simulink model "twoDOFmodel_side_wind_gust"  (R2020b)
settings: Solver=ode5  StartTime=0.0  StopTime=tf  FixedStep=dt  RelTol=1e-3
values from neighbouring files (symbols this model uses):
  I = 2500    [bicyclemodle_setp_disturbance_force_Param.m]    (also in bicyclemodle_stepParam.m; twoDOFmodel_side_wind_gust_Param.m)
  lw = -0.30    (= -0.3)    [twoDOFmodel_side_wind_gust_Param.m]
  m = 1500    [bicyclemodle_setp_disturbance_force_Param.m]    (also in bicyclemodle_stepParam.m; twoDOFmodel_side_wind_gust_Param.m)
  V = 80/3.6    (= 22.2222222222)    [bicyclemodle_setp_disturbance_force_Param.m]    (also in bicyclemodle_stepParam.m = 38.8888888889; twoDOFmodel_side_wind_gust_Param.m = 40)
  Yw = cy*0.5*p*s*(V*V+v*v)    (= 2066.58)    [twoDOFmodel_side_wind_gust_Param.m]
libraries: simulink x1
settings Model: Creator=Anson  LastModifiedBy=Anson

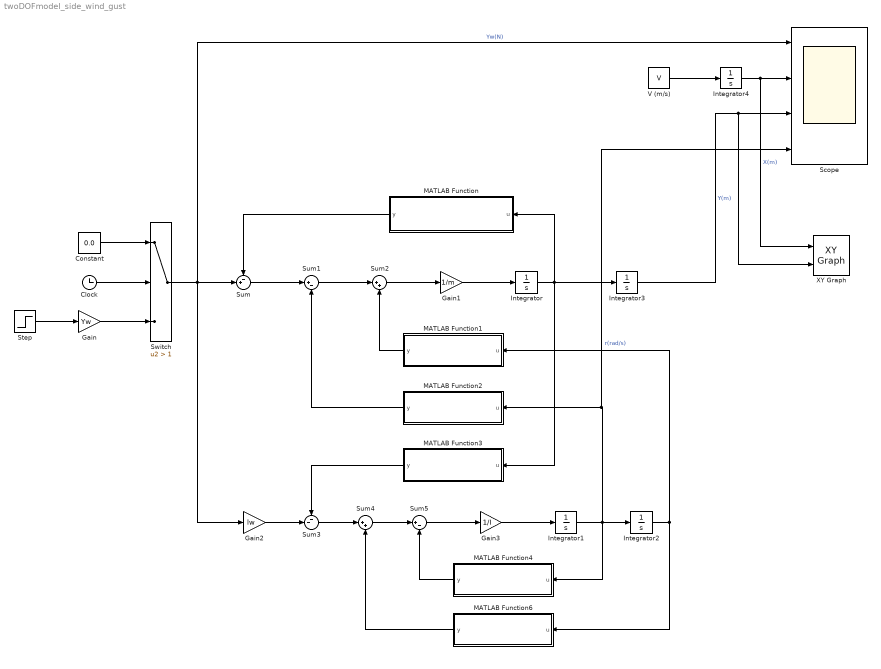
== system twoDOFmodel_side_wind_gust ==
  Clock : Clock
  Constant : Constant  Value=0.0
  Gain : Gain  Gain=Yw
  Gain1 : Gain  Gain=1/m
  Gain2 : Gain  Gain=lw
  Gain3 : Gain  Gain=1/I
  Integrator{,1..4} (5 alike) : Integrator
  MATLAB Function : MATLAB Function  TreatAsAtomicUnit=on
  MATLAB Function1 : MATLAB Function  TreatAsAtomicUnit=on
  MATLAB Function2 : MATLAB Function  TreatAsAtomicUnit=on
  MATLAB Function3 : MATLAB Function  TreatAsAtomicUnit=on
  MATLAB Function4 : MATLAB Function  TreatAsAtomicUnit=on
  MATLAB Function6 : MATLAB Function  TreatAsAtomicUnit=on
  Scope : Scope  NumInputPorts=4
  Step : Step  Time=0.5  SampleTime=0
  Sum : Sum  Inputs=-+|
  Sum1 : Sum  Inputs=|+-
  Sum2 : Sum  Inputs=|++
  Sum3 : Sum  Inputs=--|
  Sum4 : Sum  Inputs=|++
  Sum5 : Sum  Inputs=|+-
  Switch : Switch  Criteria=u2 > Threshold  Threshold=1
  V (m/s) : Constant  Value=V
  XY Graph : simulink/Sinks/XY Graph  xmin=-1  xmax=170  ymin=-1  ymax=3  st=-1
  wires:
  Step/1 -> Gain/1
  Clock/1 -> Switch/2
  Constant/1 -> Switch/1
  Gain/1 -> Switch/3
  Switch/1 -> Scope/1, Gain2/1, Sum/2  "Yw(N)"
  Sum1/1 -> Sum2/1
  Sum/1 -> Sum1/1
  Sum2/1 -> Gain1/1
  Gain1/1 -> Integrator/1
  Integrator/1 -> Integrator3/1, MATLAB Function3/1(u), MATLAB Function/1(u)
  MATLAB Function/1(y) -> Sum/1
  MATLAB Function1/1(y) -> Sum2/2
  MATLAB Function2/1(y) -> Sum1/2
  Gain2/1 -> Sum3/2
  MATLAB Function3/1(y) -> Sum3/1
  Sum3/1 -> Sum4/1
  MATLAB Function6/1(y) -> Sum4/2
  Sum4/1 -> Sum5/1
  MATLAB Function4/1(y) -> Sum5/2
  Sum5/1 -> Gain3/1
  Gain3/1 -> Integrator1/1
  Integrator1/1 -> Scope/4, MATLAB Function2/1(u), MATLAB Function4/1(u), Integrator2/1  "r(rad/s)"
  Integrator2/1 -> MATLAB Function6/1(u), MATLAB Function1/1(u)
  V (m/s)/1 -> Integrator4/1
  Integrator4/1 -> XY Graph/1, Scope/2  "X(m)"
  Integrator3/1 -> XY Graph/2, Scope/3  "Y(m)"

== matlab function twoDOFmodel_side_wind_gust/MATLAB Function ==
  data: u input; y output
function y = fcn(u)
Kf = 55000; % front cornering stiffness (N/rad)
Kr = 60000; % rear cornering stiffness (N/rad)
V = 40;         % velocity (m/s)
y = (2*(Kf+Kr)/V)*u;

== matlab function twoDOFmodel_side_wind_gust/MATLAB Function2 ==
  data: u input; y output
function y = fcn(u)
Kf = 55000; % front cornering stiffness (N/rad)
Kr = 60000; % rear cornering stiffness (N/rad)
lf = 1.1;       % distance from C.O.G to front axle (m)
lr = 1.6;       % distance from C.O.G to rear axle (m)
V = 40;         % velocity (m/s)
y = ((2*(lf*Kf-lr*Kr))/V)*u;

== matlab function twoDOFmodel_side_wind_gust/MATLAB Function3 ==
  data: u input; y output
function y = fcn(u)
Kf = 55000; % front cornering stiffness (N/rad)
Kr = 60000; % rear cornering stiffness (N/rad)
lf = 1.1;       % distance from C.O.G to front axle (m)
lr = 1.6;       % distance from C.O.G to rear axle (m)
V = 40;         % velocity (m/s)
y = ((2*(lf*Kf-lr*Kr))/V)*u;

== matlab function twoDOFmodel_side_wind_gust/MATLAB Function4 ==
  data: u input; y output
function y = fcn(u)
Kf = 55000; % front cornering stiffness (N/rad)
Kr = 60000; % rear cornering stiffness (N/rad)
lf = 1.1;       % distance from C.O.G to front axle (m)
lr = 1.6;       % distance from C.O.G to rear axle (m)
V = 40;         % velocity (m/s)
y = (2*(lf*lf*Kf+lr*lr*Kr)/V)*u;

== matlab function twoDOFmodel_side_wind_gust/MATLAB Function6 ==
  data: u input; y output
function y = fcn(u)
Kf = 55000; % front cornering stiffness (N/rad)
Kr = 60000; % rear cornering stiffness (N/rad)
lf = 1.1;       % distance from C.O.G to front axle (m)
lr = 1.6;       % distance from C.O.G to rear axle (m)
y = (2*(lf*Kf-lr*Kr))*u;

== matlab function twoDOFmodel_side_wind_gust/MATLAB Function1 ==
  data: u input; y output
function y = fcn(u)
Kf = 55000; % front cornering stiffness (N/rad)
Kr = 60000; % rear cornering stiffness (N/rad)
y = 2*(Kf+Kr)*u;
